simulink model "testVolumetricEfficiency"  (R2023a)
settings: Solver=VariableStepAuto  StartTime=0.0  StopTime=10.0  RelTol=1e-3
settings Model: Creator=rafael  LastModifiedBy=rafael

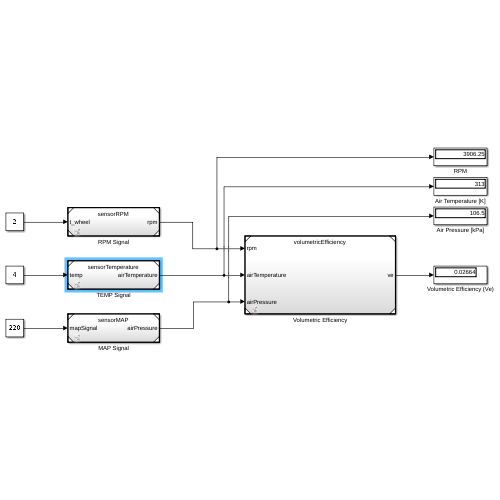
[thumbnail: Simulink's stored preview of the top-level diagram]
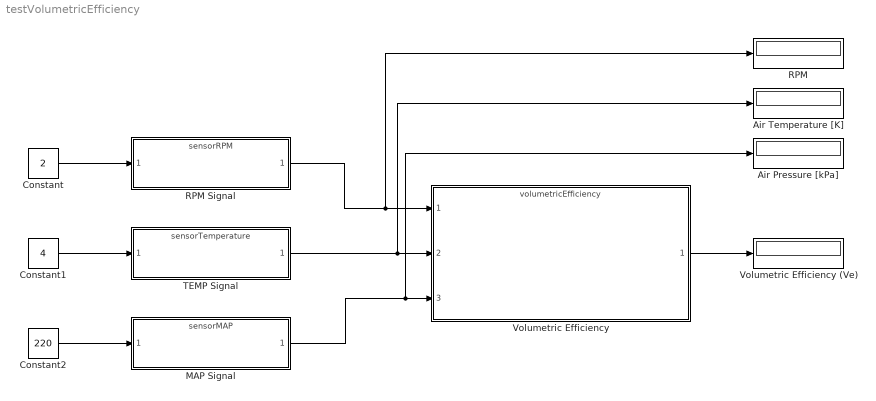
== system testVolumetricEfficiency ==
  Air Pressure [kPa] : Display
      settings: Format=decimal (Stored Integer)
  Air Temperature [K] : Display
      settings: Format=decimal (Stored Integer)
  Constant : Constant  Value=2
  Constant1 : Constant  Value=4
  Constant2 : Constant  Value=220
  MAP Signal : ModelReference  ModelNameDialog=sensorMAP.slx  SimulationMode=Normal  ModelReferenceVersion=1.3
  RPM : Display
      settings: Format=decimal (Stored Integer)
  RPM Signal : ModelReference  ModelNameDialog=sensorRPM.slx  SimulationMode=Normal  ModelReferenceVersion=1.1
  TEMP Signal : ModelReference  ModelNameDialog=sensorTemperature.slx  SimulationMode=Normal  ModelReferenceVersion=1.3
  Volumetric Efficiency : ModelReference  ModelNameDialog=volumetricEfficiency.slx  SimulationMode=Normal  ModelReferenceVersion=1.15
  Volumetric Efficiency (Ve) : Display
  wires:
  Volumetric Efficiency/1 -> Volumetric Efficiency (Ve)/1
  Constant/1 -> RPM Signal/1
  Constant2/1 -> MAP Signal/1
  Constant1/1 -> TEMP Signal/1
  MAP Signal/1 -> Volumetric Efficiency/3, Air Pressure [kPa]/1
  TEMP Signal/1 -> Air Temperature [K]/1, Volumetric Efficiency/2
  RPM Signal/1 -> RPM/1, Volumetric Efficiency/1
